simulink model "CH_humanoid_walker_rl"  (R2021a)
settings: Solver=daessc  StartTime=0.0  StopTime=params.simulation.Tf  RelTol=1e-3  AbsTol=1e-3
model workspace (MATLAB code in the model file):
  | %% Humanoid Walker With Reinforcement Learning Intialization
  | % Copyright 2019 The MathWorks, Inc.
  | 
  | %% Joint rotation limits
  | %These limits are similar to human joint rotation limits.
  | 
  | % Legs joints
  | params.jointLimits.hipFrontalUpperLimit  =  30;  % (Deg)
  | params.jointLimits.hipFrontalLowerLimit  = -90;  % (Deg)
  | params.jointLimits.kneeUpperLimit        =  90;  % (Deg)
  | params.jointLimits.kneeLowerLimit        =  5;   % (Deg)
  | params.jointLimits.ankleUpperLimit       =  20;  % (Deg)
  | params.jointLimits.ankleLowerLimit       = -20;  % (Deg)
  | % Arm joints
  | params.jointLimits.shoulderFrontalUpperLimit        =  110; % (Deg)
  | params.jointLimits.shoulderFrontalLowerLimit        = -30;  % (Deg)
  | params.jointLimits.shoulderSagittalUpperLimit       =  90;  % (Deg)
  | params.jointLimits.shoulderSagittalLowerLimit       = -30;  % (Deg)
  | params.jointLimits.elbowLowerLimit                  = 5;    % (Deg)
  | params.jointLimits.elbowUpperLimit                  = 130;  % (Deg)
  | params.jointLimits.wristLowerLimit                  = -90;  % (Deg)
  | params.jointLimits.wristUpperLimit                  = 70;   % (Deg)
  | 
  | %% Motor Parameters: Left
  | % Current motor: https://uk.rs-online.com/web/p/dc-motors/7736804
  | %Stall Torque
  | params.motor.StallTorque.LeftHip                        = 100; % (Nm)
  | params.motor.StallTorque.LeftKnee                       = 100; % (Nm)
  | params.motor.StallTorque.LeftAnkle                      = 100; % (Nm)
  | 
  | params.motor.StallTorque.LeftShoulderFrontal            = 100; % (Nm)
  | params.motor.StallTorque.LeftShoulderSagital            = 100; % (Nm)
  | params.motor.StallTorque.LeftElbow                      = 100; % (Nm)
  | params.motor.StallTorque.LeftWrist                      = 100; % (Nm)
  | 
  | %Armature Inductance: UNKNOWN
  | params.motor.ArmatureInductance.LeftHip                 = 12e-6;
  | params.motor.ArmatureInductance.LeftKnee                = 12e-6;
  | params.motor.ArmatureInductance.LeftAnkle               = 12e-6;
  | 
  | params.motor.ArmatureInductance.LeftShoulderFrontal     = 12e-6;
  | params.motor.ArmatureInductance.LeftShoulderSagital     = 12e-6;
  | params.motor.ArmatureInductance.LeftElbow               = 12e-6;
  | params.motor.ArmatureInductance.LeftWrist               = 12e-6;
  | 
  | %No-Load Speed
  | params.motor.NoLoadSpeed.LeftHip                        = 22.5; % (RPM)
  | params.motor.NoLoadSpeed.LeftKnee                       = 22.5; % (RPM)
  | params.motor.NoLoadSpeed.LeftAnkle                      = 22.5; % (RPM)
  | 
  | params.motor.NoLoadSpeed.LeftShoulderFrontal            = 22.5; % (RPM)
  | params.motor.NoLoadSpeed.LeftShoulderSagital            = 22.5; % (RPM)
  | params.motor.NoLoadSpeed.LeftElbow                      = 22.5; % (RPM)
  | params.motor.NoLoadSpeed.LeftWrist                      = 22.5; % (RPM)
  | 
  | %Torque Constant
  | params.motor.RatedDCSupply.LeftHip                      = 12; % (V)
  | params.motor.RatedDCSupply.LeftKnee                     = 12; % (V)
  | params.motor.RatedDCSupply.LeftAnkle                    = 12; % (V)
  | 
  | params.motor.RatedDCSupply.LeftShoulderFrontal          = 12; % (V)
  | params.motor.RatedDCSupply.LeftShoulderSagital          = 12; % (V)
  | params.motor.RatedDCSupply.LeftElbow                    = 12; % (V)
  | params.motor.RatedDCSupply.LeftWrist                    = 12; % (V)
  | 
  | %% Motor Parameters: Right
  | %Stall Torque
  | params.motor.StallTorque.RightHip                        = 100; % (Nm)
  | params.motor.StallTorque.RightKnee                       = 100; % (Nm)
  | params.motor.StallTorque.RightAnkle                      = 100; % (Nm)
  | 
  | params.motor.StallTorque.RightShoulderFrontal            = 100; % (Nm)
  | params.motor.StallTorque.RightShoulderSagital            = 100; % (Nm)
  | params.motor.StallTorque.RightElbow                      = 100; % (Nm)
  | params.motor.StallTorque.RightWrist                      = 100; % (Nm)
  | 
  | %Armature Inductance
  | params.motor.ArmatureInductance.RightHip                 = 12e-6;
  | params.motor.ArmatureInductance.RightKnee                = 12e-6;
  | params.motor.ArmatureInductance.RightAnkle               = 12e-6;
  | 
  | params.motor.ArmatureInductance.RightShoulderFrontal     = 12e-6;
  | params.motor.ArmatureInductance.RightShoulderSagital     = 12e-6;
  | params.motor.ArmatureInductance.RightElbow               = 12e-6;
  | params.motor.ArmatureInductance.RightWrist               = 12e-6;
  | 
  | %No-Load Speed
  | params.motor.NoLoadSpeed.RightHip                        = 22.5; % (RPM)
  | params.motor.NoLoadSpeed.RightKnee                       = 22.5; % (RPM)
  | params.motor.NoLoadSpeed.RightAnkle                      = 22.5; % (RPM)
  | 
  | params.motor.NoLoadSpeed.RightShoulderFrontal            = 22.5; % (RPM)
  | params.motor.NoLoadSpeed.RightShoulderSagital            = 22.5; % (RPM)
  | params.motor.NoLoadSpeed.RightElbow                      = 22.5; % (RPM)
  | params.motor.NoLoadSpeed.RightWrist                      = 22.5; % (RPM)
  | 
  | %Torque Constant
  | params.motor.RatedDCSupply.RightHip                      = 12; % (V)
  | params.motor.RatedDCSupply.RightKnee                     = 12; % (V)
  | params.motor.RatedDCSupply.RightAnkle                    = 12; % (V)
  | 
  | params.motor.RatedDCSupply.RightShoulderFrontal          = 12; % (V)
  | params.motor.RatedDCSupply.RightShoulderSagital          = 12; % (V)
  | params.motor.RatedDCSupply.RightElbow                    = 12; % (V)
  | params.motor.RatedDCSupply.RightWrist                    = 12; % (V)
  | 
  | 
  | %% Material properties
  | 
  | params.materialProperties.lowerBodyDensity = 990;  % (kg/m^3)
  | params.materialProperties.upperBodyDensity = 1900; % (kg/m^3)
  | 
  | %% World damping
  | % We add damping to the vertical (z) and rotational (Rx, Ry, Rz) components
  | % of the bushing joint. This dissipates energy from the system and facilates
  | % quicker learning. Increasing this improves stability and learning, but is
  | % less realistic.
  | 
  | params.simulation.worldDamping = 6; % (Ns/m)
  | 
  | %% Simulation parameters
  | 
  | params.simulation.initialHeight=1.54; % (m) Intial height of robot
  | params.simulation.Ts = 0.025;         % (s) Control and sensing discretization time
  | params.simulation.Tf = 600;      % (s) Max simulation time
  | 
  | %% Spatial contact force block parameters.
  | % The value of these parameters affects simulation and learning speed.
  | % Higher damping generally improves learning but slows down simulation.
  | % High static and dynamic friction values tend to improve learning.
  | 
  | params.contact.stiffness        = 1e5;  % (N/m)
  | params.contact.damping          = 1e5;  % (Ns/m)
  | params.contact.transitionWidth  = 1e-3; % (m)
  | params.contact.staticFriction   = 1;    % ()
  | params.contact.dynamicFriction  = 0.9;  % ()
  | params.contact.criticalVelocity = 1e-3; % (m/s)
  | params.contact.contactRadius = 0.01;    % (m)
  | 
  | %% Controller parameters
  | 
  | params.controller.hipFrontalStiffness  = 80; % (N*m/rad)
  | params.controller.hipFrontalDamping    = 1;  % (N*m*s/rad)
  | params.controller.kneeStiffness        = 80; % (N*m*/rad)
  | params.controller.kneeDamping          = 1;  % (N*m*s/rad)
  | params.controller.ankleStiffness       = 80; % (N*m/rad)
  | params.controller.ankleDamping         = 1;  % (N*m*s/rad)
  | 
  | 
  | %% Stopping criteria
  | % Define the conditions under which the simulation is terminated early.
  | % One or more of three conditions need to be satisfied for termination.
  | % If the humanoid torso drops vertically, travels laterally or rotates in
  | % any axis more than a set of predefined values, or if the humanoid stops
  | % moving.
  | 
  | params.stoppingCriteria.heightChange     = 0.5; % (m)
  | params.stoppingCriteria.lateral          = 1000;   % (m)
  | params.stoppingCriteria.angle            = 60;  % (deg)
  | params.stoppingCriteria.timeoutTime      = 2;   % (s)
  | params.stoppingCriteria.timeoutDistance  = 1;   % (m)
  | 
  | %% Reward scaling parameters
  | 
  | params.reward.boxMoveRewardWeight   = 5;    % Object motion reward scale, w_1
  | params.reward.forwardRewardWeight   = 1;    % Forward velocity scale, w_2
  | params.reward.timestepRewardWeight  = -0.5;    % Not falling scale, w_3 - Penalise time taken, Strive to always move forward
  | params.reward.powerPenaltyWeight    = 5e-4; % Power scale, w_4
  | params.reward.verticalPenaltyWeight = 25;   % Vertical displacement scale, w_5
  | params.reward.lateralPenaltyWeight  = 2;  % Lateral displacement scale, w_6
  | 
  | %% Display parameters
  | 
  | params.display.tileColour    = [0.956, 0.941, 0.941];
  | params.display.floorColour   = [0.756, 0.741, 0.741];
  | params.display.tileThickness = 0.005;
  | params.display.planeWidth        = 100;   % (m)
  | params.display.planeLength       = 200;  % (m)
  | params.display.planeHeight       = 1;   % (m)
  | params.display.Gravity           = [0, 0, -9.80665];   % (m/s^2)
undefined symbols (not defined in the file or in its folder): Connection1, Connection2, Connection3, Connection4, Connection5, Connection6, Connection7, Connection8, rl, X, Y, Z
libraries: sm_lib x26, CH_Library x8, nesl_utility x4, rllib x1
settings Model: Creator=The MathWorks, Inc.  LastModifiedBy=coa19cdd
settings SolverCC: AlgebraicLoopSolver=TrustRegion
settings DebuggingCC: ParameterPrecisionLossMsg=none  ParameterTunabilityLossMsg=none  SFMachineParentedDataDiag=warning
settings ExplorerConfigSet: InternalSimMechanicsExplorerSettings="<ExplorerConfiguration><canonicalview>default</canonicalview><AnimationSetting><BasePlaybackSpeed>1.0</BasePlaybackSpeed><PlaybackSpeedFactor>1.0</PlaybackSpeedFactor></AnimationSetting><TilePanel><TileInfo><Tiles Columns=\"1\" Count=\"1\" Rows=\"1\"><Column Weight=\"1\"/><Row Weight=\"1\"/><Tile Height=\"1\" Width=\"1\" X=\"0\" Y=\"0\"/></Tiles></TileInfo><SceneInfo><SceneViewer><BGColor><R>0.800000011920928955</R><G>1</G><B>1</B></BGColor><Camera><DoPerspective>on</DoPerspective><Position><X>41.8085971876439402</X><Y>-114.741449940210288</Y><Z>43.3892163501630179</Z></Position><Center><X>-86.6397285289506698</X><Y>13.7068757763843223</Y><Z>-85.0591093664316418</Z></Center><Up><X>-0.408248290463863073</X><Y>0.408248290463863073</Y><Z>0.816496580927726145</Z></Up><ViewLimDist>1</ViewLimDist><YLim>0.466307658154998583</YLim><XLim>0.727439946721797792</XLim></Camera></SceneViewer></SceneInfo></TilePanel><MechEditorPanel><Cameras><Camera><Id>Camera1</Id><Value><Name>Camera1</Name><NativeCamera><PositionTrackingFeature>Humanoid_Walker.Humanoid_Robot_6_Joint.Camera_Frame.R</PositionTrackingFeature><CenterTrackingFeature>Humanoid_Walker.Humanoid_Robot_6_Joint.Aim_Frame.R</CenterTrackingFeature><UpVectorTrackingFeature>Humanoid_Walker.Humanoid_Robot_6_Joint.World.W</UpVectorTrackingFeature><CenterTrackingOrigin>on</CenterTrackingOrigin><UpVectorTrackingDirection>+Z</UpVectorTrackingDirection></NativeCamera></Value></Camera></Cameras><GfxPanelCameraMap><MapElement CameraMLId=\"Camera1\" GfxPanelIndex=\"0\"/></GfxPanelCameraMap><VideoCreator><PlaybackSpeedRatio>1.0</PlaybackSpeedRatio><FrameRate>30</FrameRate><VideoFormat>Motion JPEG AVI</VideoFormat><FrameSize>auto</FrameSize></VideoCreator></MechEditorPanel></ExplorerConfiguration>"

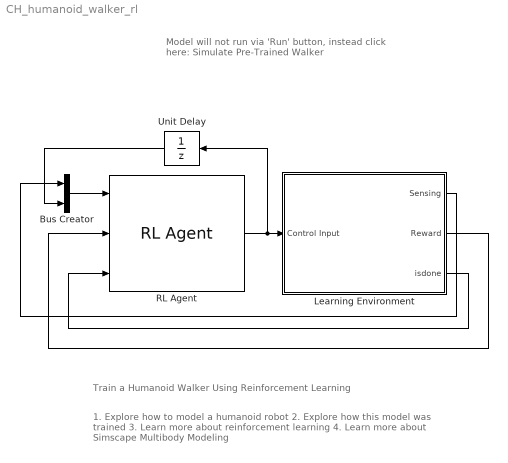
== system CH_humanoid_walker_rl ==
  note: Train a Humanoid Walker Using Reinforcement Learning
  note: Model will not run via 'Run' button, instead click here:
      | Simulate Pre-Trained Walker
  note: 1. Explore how to model a humanoid robot
      | 2. Explore how this model was trained
      | 3. Learn more about reinforcement learning
      | 4. Learn more about Simscape Multibody Modeling
  Bus Creator : BusCreator  Inputs=2
  Learning Environment : Subsystem
  RL Agent : rllib/RL Agent  Agent=rl.util.PolicyInstance.get()  ExternalActionAsInput=off  ProvideCumRwd=off  TreatAsDirectFeedthrough=on
  Unit Delay : UnitDelay  SampleTime=params.simulation.Ts  HasFrameUpgradeWarning=on
  wires:
  RL Agent/1 -> Unit Delay/1, Learning Environment/1(Control Input)
  Learning Environment/2("Reward ") -> RL Agent/2
  Learning Environment/3(isdone) -> RL Agent/3
  Bus Creator/1 -> RL Agent/1
  Unit Delay/1 -> Bus Creator/2
  Learning Environment/1(Sensing) -> Bus Creator/1

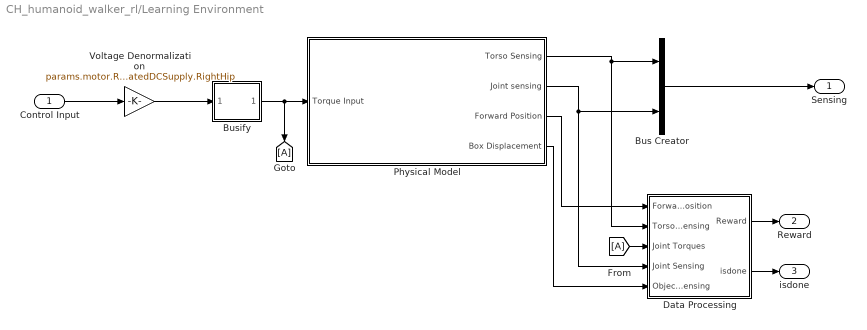
== system CH_humanoid_walker_rl/Learning Environment ==
  Control Input : Inport
  Bus Creator : BusCreator  Inputs=2
  Busify : Subsystem
  Data Processing : Subsystem
  Physical Model : Subsystem
  Voltage Denormalization : Gain  Gain=params.motor.RatedDCSupply.RightHip
  Sensing : Outport
  "Reward " : Outport  Port=2
  isdone : Outport  Port=3
  wires:
  Control Input/1 -> Voltage Denormalization/1
  Physical Model/1(Torso Sensing) -> Data Processing/2(Torso Sensing), Bus Creator/1
  Physical Model/2(Joint sensing) -> Data Processing/4(Joint Sensing), Bus Creator/2
  Busify/1(Out1) -> [A], Physical Model/1(Torque Input)
  [A] -> Data Processing/3(Joint Torques)
  Data Processing/1(Reward) -> "Reward "/1
  Data Processing/2(isdone) -> isdone/1
  Physical Model/3(Forward Position) -> Data Processing/1(Forward Position)
  Voltage Denormalization/1 -> Busify/1(Control Input)
  Bus Creator/1 -> Sensing/1
  Physical Model/4(Box Displacement) -> Data Processing/5(Object Sensing)

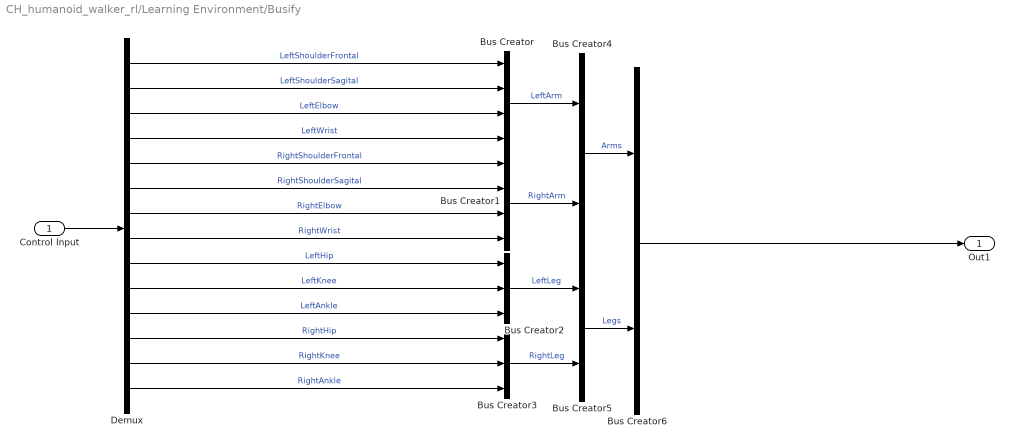
== system CH_humanoid_walker_rl/Learning Environment/Busify ==
  Control Input : Inport
  Bus Creator : BusCreator  Inputs=4
  Bus Creator1 : BusCreator  Inputs=4
  Bus Creator2 : BusCreator  Inputs=3
  Bus Creator3 : BusCreator  Inputs=3
  Bus Creator4 : BusCreator  Inputs=2
  Bus Creator5 : BusCreator  Inputs=2
  Bus Creator6 : BusCreator  Inputs=2
  Demux : Demux  Outputs=14
  Out1 : Outport
  wires:
  Control Input/1 -> Demux/1
  Demux/1 -> Bus Creator/1  "LeftShoulderFrontal"
  Demux/2 -> Bus Creator/2  "LeftShoulderSagital"
  Demux/3 -> Bus Creator/3  "LeftElbow"
  Demux/4 -> Bus Creator/4  "LeftWrist"
  Demux/5 -> Bus Creator1/1  "RightShoulderFrontal"
  Demux/6 -> Bus Creator1/2  "RightShoulderSagital"
  Demux/7 -> Bus Creator1/3  "RightElbow"
  Demux/8 -> Bus Creator1/4  "RightWrist"
  Demux/9 -> Bus Creator2/1  "LeftHip"
  Demux/10 -> Bus Creator2/2  "LeftKnee"
  Demux/11 -> Bus Creator2/3  "LeftAnkle"
  Demux/12 -> Bus Creator3/1  "RightHip"
  Demux/13 -> Bus Creator3/2  "RightKnee"
  Demux/14 -> Bus Creator3/3  "RightAnkle"
  Bus Creator/1 -> Bus Creator4/1  "LeftArm"
  Bus Creator1/1 -> Bus Creator4/2  "RightArm"
  Bus Creator2/1 -> Bus Creator5/1  "LeftLeg"
  Bus Creator3/1 -> Bus Creator5/2  "RightLeg"
  Bus Creator4/1 -> Bus Creator6/1  "Arms"
  Bus Creator5/1 -> Bus Creator6/2  "Legs"
  Bus Creator6/1 -> Out1/1

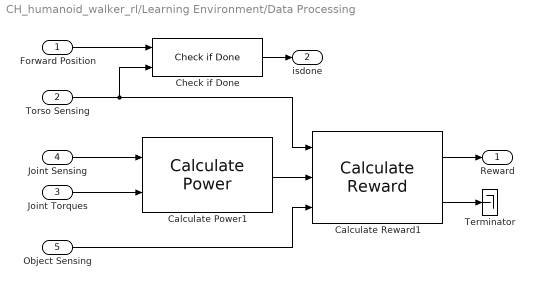
== system CH_humanoid_walker_rl/Learning Environment/Data Processing ==
  Forward Position : Inport
  Torso Sensing : Inport  Port=2
  Joint Torques : Inport  Port=3
  Joint Sensing : Inport  Port=4
  Object Sensing : Inport  Port=5
  Calculate Power1 : CH_Library/Calculate Power  SystemSampleTime=-1  VariantActivationTime=update diagram  Latency=0  AutoFrameSizeCalculation=off
  Calculate Reward1 : CH_Library/Calculate Reward  BoxReward=params.reward.boxMoveRewardWeight  forwardReward=params.reward.forwardRewardWeight  timestepReward=params.reward.timestepRewardWeight  powerPenalty=params.reward.powerPenaltyWeight  verticalPenalty=params.reward.verticalPenaltyWeight  lateralPenalty=params.reward.lateralPenaltyWeight
  Check if Done : CH_Library/Check if Done  verticalStop=params.stoppingCriteria.heightChange  lateralStop=params.stoppingCriteria.lateral  angularStop=params.stoppingCriteria.angle  timeoutTime=params.stoppingCriteria.timeoutTime  timeoutDistance=params.stoppingCriteria.timeoutDistance
  Terminator : Terminator
  Reward : Outport
  isdone : Outport  Port=2
  wires:
  Torso Sensing/1 -> Calculate Reward1/1, Check if Done/2
  Check if Done/1 -> isdone/1
  Calculate Power1/1 -> Calculate Reward1/2
  Joint Sensing/1 -> Calculate Power1/1
  Joint Torques/1 -> Calculate Power1/2
  Calculate Reward1/1 -> Reward/1
  Forward Position/1 -> Check if Done/1
  Calculate Reward1/2 -> Terminator/1
  Object Sensing/1 -> Calculate Reward1/3

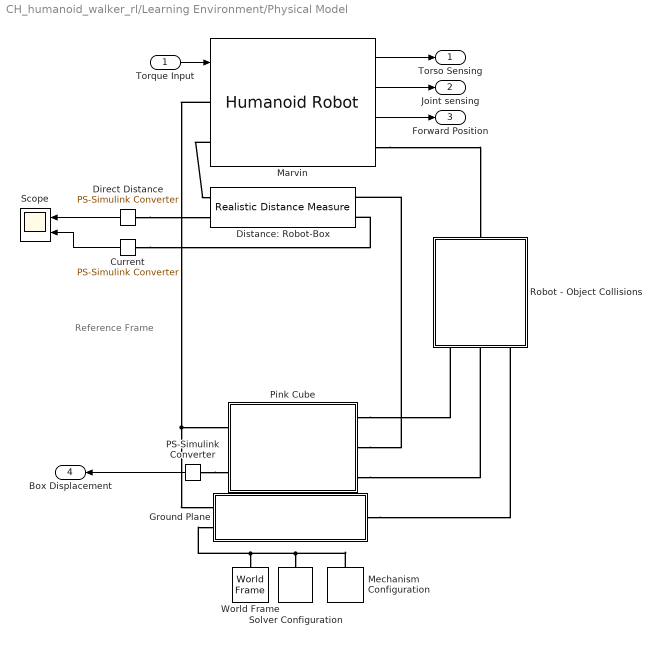
== system CH_humanoid_walker_rl/Learning Environment/Physical Model ==
  note: Reference Frame
  Torque Input : Inport
  Current : nesl_utility/PS-Simulink Converter  PhysicalDomain=network_engine_domain  SubClassName=ps_output  LeftPortType=input  RightPortType=output  PseudoPeriodic=off  Frequencies=[]  Unit=inherit  AffineConversion=off
      settings: SourceProductBaseCode=PW,SS
  Direct Distance : nesl_utility/PS-Simulink Converter  PhysicalDomain=network_engine_domain  SubClassName=ps_output  LeftPortType=input  RightPortType=output  PseudoPeriodic=off  Frequencies=[]  Unit=inherit  AffineConversion=off
      settings: SourceProductBaseCode=PW,SS
  Distance: Robot-Box : CH_Library/Realistic Distance Measure  LEDC=1.0
  Ground Plane : Subsystem
  Marvin : CH_Library/Humanoid Robot  contactRadius=params.contact.contactRadius  contactStiffness=params.contact.stiffness  contactDamping=params.contact.damping  contactTWidth=params.contact.transitionWidth  contactStaticFriction=params.contact.staticFriction  contactDynamicFriction=params.contact.dynamicFriction  contactCriticalVelocity=params.contact.criticalVelocity  footDensity=params.materialProperties.lowerBodyDensity  lowerLegDensity=params.materialProperties.lowerBodyDensity  upperLegDensity=params.materialProperties.lowerBodyDensity  hipDensity=params.materialProperties.lowerBodyDensity  trunkDensity=params.materialProperties.upperBodyDensity  shoulderDensity=params.materialProperties.upperBodyDensity  upperArmDensity=params.materialProperties.upperBodyDensity  lowerArmDensity=params.materialProperties.upperBodyDensity  handDensity=params.materialProperties.upperBodyDensity  headDensity=params.materialProperties.upperBodyDensity  hipUpperLimit=params.jointLimits.hipFrontalUpperLimit  hipLowerLimit=params.jointLimits.hipFrontalLowerLimit  kneeUpperLimit=params.jointLimits.kneeUpperLimit  kneeLowerLimit=params.jointLimits.kneeLowerLimit  ankleUpperLimit=params.jointLimits.ankleUpperLimit  ankleLowerLimit=params.jointLimits.ankleLowerLimit  shoulderFrontalUpperLimit=params.jointLimits.shoulderFrontalUpperLimit  shoulderFrontalLowerLimit=params.jointLimits.shoulderFrontalLowerLimit  shoulderSagittalUpperLimit=params.jointLimits.shoulderSagittalUpperLimit  shoulderSagittalLowerLimit=params.jointLimits.shoulderSagittalLowerLimit  elbowUpperLimit=params.jointLimits.ankleUpperLimit  elbowLowerLimit=params.jointLimits.shoulderSagittalLowerLimit  wristUpperLimit=params.jointLimits.ankleUpperLimit  wristLowerLimit=params.jointLimits.shoulderSagittalLowerLimit
      link override Torso and Head/Camera: Y_TF=5.0  X_ROT=10
  Mechanism Configuration : sm_lib/Utilities/Mechanism Configuration  UniformGravity=Constant  GravityVector=[0, 0, -9.80665]  GravityVectorUnits=m/s^2  GravityUnits=m/s^2  LinearizationDelta=0.001  JointModeTransitionNonlinearIterations=2
  PS-Simulink Converter : nesl_utility/PS-Simulink Converter  PhysicalDomain=network_engine_domain  SubClassName=ps_output  LeftPortType=input  RightPortType=output  PseudoPeriodic=off  Frequencies=[]  Unit=inherit  AffineConversion=off
      settings: SourceProductBaseCode=PW,SS
  Pink Cube : Subsystem  AncestorBlock=CH_Library/Brick Object Hybrid  mask{BW=1, BDep=1, BH=1, XDis=0, YDis=3, ZDis=0.6, XRot=0, YRot=0, ZRot=0, BDen=5, BlockRed=1.0, BlockGreen=0.680, BlockBlue=0.710, BlockOpac=1}
      mask prompts: BW "Width (X)"; BDep "Depth (Y)"; BH "Height (Z)"; XDis "X Displacement"; YDis "Y Displacement"; ZDis "Z Displacement"; XRot "Rotation about X"; YRot "Rotation about Y"; ZRot "Rotation about Z"; BDen "Density"; BlockRed "Red tint"; BlockGreen "Green tint"; BlockBlue "Blue tint"; BlockOpac "Opacity"
      mask DialogControl Container8 Prompt: Block Dimensions
      mask DialogControl Container11 Prompt: Block Placement
      mask DialogControl Container14 Prompt: Block Rotation
      mask DialogControl Control1 Prompt: Rotations completed in sequence: X,Y,Z
      mask DialogControl Container5 Prompt: Block Properties
  Robot - Object Collisions : Subsystem
      settings: PortSchema="{\"entries\":[{\"content\":{\"sides\":[{\"content\":{\"connectorIds\":[]},\"type\":\"ConnectorPlacement.EquallySpacedRectSide\",\"uuid\":\"b00614a5-f09e-422d-bac9-77beaa757f34\"},{\"content\":{\"connectorIds\":[],\"side\":\"RIGHT\"},\"type\":\"ConnectorPlacement.EquallySpacedRectSide\",\"uuid\":\"f8121b2f-8181-47c9-add5-f5a413d142f6\"},{\"content\":{\"connectorIds\":[\"LConn1\"],\"side\":\"TOP\"},\"type\":\"ConnectorPlacement.EquallySpacedRectSide\",\"uuid\":\"8b595efc-2aff-4bc7-847e-9a9432c1292e\"},{\"content\":{\"connectorIds\":[\"RConn1\",\"RConn2\",\"RConn3\"],\"side\":\"BOTTOM\"},\"type\":\"ConnectorPlacement.EquallySpacedRectSide\",\"uuid\":\"30d4c700-0653-4c9a-a829-31e4e720a8eb\"}]},\"type\":\"ConnectorPlacement.EquallySpacedConnector\",\"uuid\":\"6d11a0b2-f15b-484e-9b2d-8ecd8f664af7\"}],\"packageUris\":[\"http://schema.mathworks.com/mf0/Connector/R2020b\"],\"version\":\"1.0\"}"
  Scope : Scope  NumInputPorts=2
  Solver Configuration : nesl_utility/Solver Configuration  PhysicalDomain=network_engine_domain  SubClassName=solver  LeftPortType=input  RightPortType=generic  Tones=[]  Harmonics=[]  SimulateNoise=off  Profile=off  UseLocalSampling=off  EnableSwitchedLinearOptims=on  FrequencyDomain=off  UseCCode=off  RelTol=0.001  AbsTol=1e-06  MinStep=1e-09  ToWorkspace=off  RevertToSquareIcSolve=off  NumHomotopyIterations=100  PhasorMode=off  PhasorModeNumHarmonics=1  DoDC=off  ResidualTolerance=1e-09  UseLocalSolver=off  LocalSolverChoice=NE_BACKWARD_EULER_ADVANCER  LocalSolverSampleTime=0.001  DoFixedCost=off  MaxNonlinIter=3  MaxModeIter=2  ComputeImpulses=off  ImpulseIterations=2  LinearAlgebra=auto  EquationFormulation=NE_TIME_EF  DelaysMemoryBudget=1024  AutomaticFiltering=on  FilteringTimeConstant=0.001  PartitionStorageMethod=AS_NEEDED  PartitionMemoryBudget=1024  PartitionMethod=ROBUST
      settings: SourceProductBaseCode=PW,SS
  World Frame : sm_lib/Frames and Transforms/World Frame
  Torso Sensing : Outport
  Joint sensing : Outport  Port=2
  Forward Position : Outport  Port=3
  Box Displacement : Outport  Port=4
  wires:
  Torque Input/1 -> Marvin/1
  Marvin/3 -> Forward Position/1
  Marvin/2 -> Joint sensing/1
  Marvin/1 -> Torso Sensing/1
  Current/1 -> Scope/2
  Direct Distance/1 -> Scope/1
  PS-Simulink Converter/1 -> Box Displacement/1
  connections:
  Mechanism Configuration/RConn1 -- World Frame/RConn1 -- Ground Plane/LConn2 -- Solver Configuration/RConn1
  Marvin/LConn1 -- Pink Cube/LConn1 -- Ground Plane/LConn1
  Marvin/LConn2 -- Distance: Robot-Box/LConn1
  Pink Cube/RConn2 -- Distance: Robot-Box/RConn1
  Current/LConn1 -- Distance: Robot-Box/RConn2
  Direct Distance/LConn1 -- Distance: Robot-Box/LConn2
  Marvin/RConn1 -- Robot - Object Collisions/LConn1
  Ground Plane/RConn1 -- Robot - Object Collisions/RConn3
  Pink Cube/RConn1 -- Robot - Object Collisions/RConn1
  PS-Simulink Converter/LConn1 -- Pink Cube/LConn2
  Pink Cube/RConn3 -- Robot - Object Collisions/RConn2

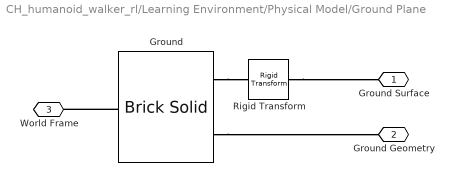
== system CH_humanoid_walker_rl/Learning Environment/Physical Model/Ground Plane ==
  Ground : sm_lib/Body Elements/Brick Solid  GraphicAmbientColor=[0.15 0.15 0.15 1.0]  BasedOnType=Density  BrickDimensions=[params.display.planeWidth params.display.planeLength params.display.planeHeight]  BrickDimensionUnits=m  CenterOfMass=[0 0 0]  CenterOfMassUnits=m  GraphicDiffuseColor=params.display.floorColour  Density=1000  DensityUnits=kg/m^3  DoExposeReferenceFrame=on  GraphicEmissiveColor=[0.0 0.0 0.0 1.0]  ExportEntireGeometry=on  SerializedFrames=<Frames><Frame><Id>Frame1</Id><Value><Name>GS</Name><Origin><Source>GeometricFeature</Source><FeatureName>+z surface</FeatureName></Origin><PrimaryAxis><DefinedDirection>+Z</DefinedDirection><Source>ReferenceFrame</Source><SourceDirection>+Z</SourceDirection><FeatureName></FeatureName></PrimaryAxis><SecondaryAxis><DefinedDirection>+X</DefinedDirection><Source>ReferenceFrame</Source><SourceDirection>+X</SourceDirection><FeatureName></FeatureName></SecondaryAxis></Value></Frame></Frames>  MarkerShape=Sphere  MarkerSize=10  GraphicType=FromGeometry  InertiaType=CalculateFromGeometry  Mass=1  MassUnits=kg  MomentsOfInertia=[1 1 1]  MomentsOfInertiaUnits=kg*m^2  GraphicOpacity=0.3  ProductsOfInertia=[0 0 0]  ProductsOfInertiaUnits=kg*m^2  GraphicShininess=75  GraphicSpecularColor=[0.5 0.5 0.5 1.0]  GraphicVisPropType=SimpleVisualProperties
  Rigid Transform : sm_lib/Frames and Transforms/Rigid Transform  TranslationMethod=StandardAxis  TranslationStandardOffset=0.5-(params.display.planeLength/2)  TranslationLengthUnit=m  TranslationStandardAxis=+Y  TranslationCartesianOffset=[0 0 0]  TranslationROffset=0  TranslationROffsetUnits=m  TranslationZOffset=0  TranslationZOffsetUnits=m  TranslationThetaOffset=0  TranslationThetaOffsetUnits=deg  RotationMethod=None  RotationAngleUnits=deg  RotationStandardAxis=+Z  RotationAngle=0.0  RotationArbitraryAxis=[0 0 1]  FollAlignAxisA=+X  BaseAlignAxisA=+Y  FollAlignAxisB=+Y  BaseAlignAxisB=+Z  RotationSequenceAxes=FollowerAxes  RotationSequence=XYX  RotationSequenceAngles=[0 0 0]  RotationSequenceAnglesUnits=deg  RotationMatrix=[1 0 0; 0 1 0; 0 0 1]
  Ground Surface : PMIOPort  Side=Left
  Ground Geometry : PMIOPort  Port=2  Side=Right
  World Frame : PMIOPort  Port=3  Side=Left
  connections:
  Ground/LConn1 -- Rigid Transform/LConn1
  Ground/LConn2 -- Ground Geometry/RConn1
  Ground/RConn1 -- World Frame/RConn1
  Rigid Transform/RConn1 -- Ground Surface/RConn1

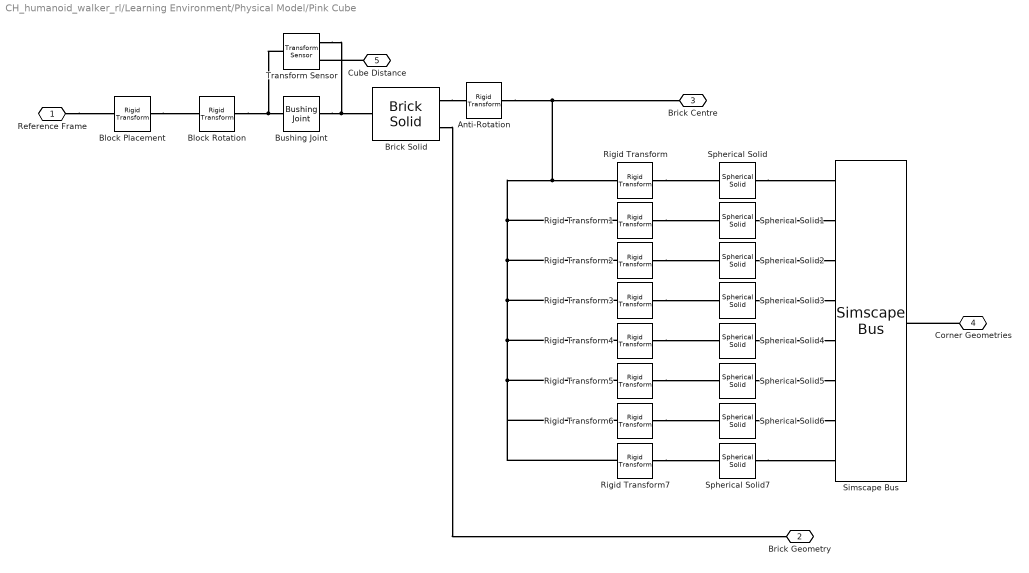
== system CH_humanoid_walker_rl/Learning Environment/Physical Model/Pink Cube ==
  Anti-Rotation : sm_lib/Frames and Transforms/Rigid Transform  TranslationMethod=None  TranslationStandardOffset=0  TranslationLengthUnit=m  TranslationStandardAxis=+Z  TranslationCartesianOffset=[0 0 0]  TranslationROffset=0  TranslationROffsetUnits=m  TranslationZOffset=0  TranslationZOffsetUnits=m  TranslationThetaOffset=0  TranslationThetaOffsetUnits=deg  RotationMethod=RotationSequence  RotationAngleUnits=deg  RotationStandardAxis=+Z  RotationAngle=0.0  RotationArbitraryAxis=[0 0 1]  FollAlignAxisA=+X  BaseAlignAxisA=+Y  FollAlignAxisB=+Y  BaseAlignAxisB=+Z  RotationSequenceAxes=BaseAxes  RotationSequence=XYZ  RotationSequenceAngles=[-XRot -YRot -ZRot]  RotationSequenceAnglesUnits=deg  RotationMatrix=[1 0 0; 0 1 0; 0 0 1]
  Block Placement : sm_lib/Frames and Transforms/Rigid Transform  TranslationMethod=Cartesian  TranslationStandardOffset=0  TranslationLengthUnit=m  TranslationStandardAxis=+Z  TranslationCartesianOffset=[XDis YDis ZDis]  TranslationROffset=0  TranslationROffsetUnits=m  TranslationZOffset=0  TranslationZOffsetUnits=m  TranslationThetaOffset=0  TranslationThetaOffsetUnits=deg  RotationMethod=None  RotationAngleUnits=deg  RotationStandardAxis=+Z  RotationAngle=0.0  RotationArbitraryAxis=[0 0 1]  FollAlignAxisA=+X  BaseAlignAxisA=+Y  FollAlignAxisB=+Y  BaseAlignAxisB=+Z  RotationSequenceAxes=FollowerAxes  RotationSequence=XYX  RotationSequenceAngles=[0 0 0]  RotationSequenceAnglesUnits=deg  RotationMatrix=[1 0 0; 0 1 0; 0 0 1]
  Block Rotation : sm_lib/Frames and Transforms/Rigid Transform  TranslationMethod=None  TranslationStandardOffset=0  TranslationLengthUnit=m  TranslationStandardAxis=+Z  TranslationCartesianOffset=[0 0 0]  TranslationROffset=0  TranslationROffsetUnits=m  TranslationZOffset=0  TranslationZOffsetUnits=m  TranslationThetaOffset=0  TranslationThetaOffsetUnits=deg  RotationMethod=RotationSequence  RotationAngleUnits=deg  RotationStandardAxis=+Z  RotationAngle=0.0  RotationArbitraryAxis=[0 0 1]  FollAlignAxisA=+X  BaseAlignAxisA=+Y  FollAlignAxisB=+Y  BaseAlignAxisB=+Z  RotationSequenceAxes=BaseAxes  RotationSequence=XYZ  RotationSequenceAngles=[XRot YRot ZRot]  RotationSequenceAnglesUnits=deg  RotationMatrix=[1 0 0; 0 1 0; 0 0 1]
  Brick Solid : sm_lib/Body Elements/Brick Solid  GraphicAmbientColor=[0.15 0.15 0.15 1.0]  BasedOnType=Density  BrickDimensions=[BW BDep BH]  BrickDimensionUnits=m  CenterOfMass=[0 0 0]  CenterOfMassUnits=m  GraphicDiffuseColor=[BlockRed BlockGreen BlockBlue]  Density=BDen  DensityUnits=kg/m^3  DoExposeReferenceFrame=on  GraphicEmissiveColor=[0.0 0.0 0.0 1.0]  ExportEntireGeometry=on  SerializedFrames=<Frames><Frame><Id>Frame1</Id><Value><Name>Block Centre</Name><Origin><Source>ReferenceFrame</Source><FeatureName></FeatureName></Origin><PrimaryAxis><DefinedDirection>+Z</DefinedDirection><Source>ReferenceFrame</Source><SourceDirection>+Z</SourceDirection><FeatureName></FeatureName></PrimaryAxis><SecondaryAxis><DefinedDirection>+X</DefinedDirection><Source>ReferenceFrame</Source><SourceDirection>+X</SourceDirection><FeatureName></FeatureName></SecondaryAxis></Value></Frame></Frames>  MarkerShape=Sphere  MarkerSize=10  GraphicType=FromGeometry  InertiaType=CalculateFromGeometry  Mass=1  MassUnits=kg  MomentsOfInertia=[1 1 1]  MomentsOfInertiaUnits=kg*m^2  GraphicOpacity=BlockOpac  ProductsOfInertia=[0 0 0]  ProductsOfInertiaUnits=kg*m^2  GraphicShininess=75  GraphicSpecularColor=[0.5 0.5 0.5 1.0]  GraphicVisPropType=SimpleVisualProperties
  Bushing Joint : sm_lib/Joints/Bushing Joint  JointMode=Normal  SenseConstraintForce=off  SenseConstraintForceX=off  SenseConstraintForceY=off  SenseConstraintForceZ=off  SenseConstraintTorque=off  SenseConstraintTorqueX=off  SenseConstraintTorqueY=off  SenseConstraintTorqueZ=off  SenseTotalForce=off  SenseTotalForceX=off  SenseTotalForceY=off  SenseTotalForceZ=off  SenseTotalTorque=off  SenseTotalTorqueX=off  SenseTotalTorqueY=off  SenseTotalTorqueZ=off  CompositeWrenchDir=FollowerOnBase  CompositeWrenchFrame=BaseFrame  PxEquilibriumPosition=0  PxEquilibriumPositionUnits=m  PxSpringStiffness=0  PxSpringStiffnessUnits=N/m  PxDampingCoefficient=0  PxDampingCoefficientUnits=N/(m/s)  PxTorqueActuationMode=NoTorque  PxMotionActuationMode=ComputedMotion  PxSensePosition=off  PxSenseVelocity=off  PxSenseAcceleration=off  PxSenseTorqueForce=off  PxSenseLowerLimitTorqueForce=off  PxSenseUpperLimitTorqueForce=off  PxLowerLimitSpecify=off  PxLowerLimitBound=-1  PxLowerLimitBoundUnits=m  PxLowerLimitStiffness=1e6  PxLowerLimitStiffnessUnits=N/m  PxLowerLimitDamping=1e3  PxLowerLimitDampingUnits=N/(m/s)  PxLowerLimitTransitionRegionWidth=1e-4  PxLowerLimitTransitionRegionWidthUnits=m  PxUpperLimitSpecify=off  PxUpperLimitBound=1  PxUpperLimitBoundUnits=m  PxUpperLimitStiffness=1e6  PxUpperLimitStiffnessUnits=N/m  PxUpperLimitDamping=1e3  PxUpperLimitDampingUnits=N/(m/s)  PxUpperLimitTransitionRegionWidth=1e-4  PxUpperLimitTransitionRegionWidthUnits=m  PxPositionTargetSpecify=off  PxPositionTargetPriority=High  PxPositionTargetValue=0  PxPositionTargetValueUnits=m  PxVelocityTargetSpecify=off  PxVelocityTargetPriority=High  PxVelocityTargetValue=0  PxVelocityTargetValueUnits=m/s  PyEquilibriumPosition=0  PyEquilibriumPositionUnits=m  PySpringStiffness=0  PySpringStiffnessUnits=N/m  PyDampingCoefficient=0  PyDampingCoefficientUnits=N/(m/s)  PyTorqueActuationMode=NoTorque  PyMotionActuationMode=ComputedMotion  PySensePosition=off  PySenseVelocity=off  PySenseAcceleration=off  PySenseTorqueForce=off  PySenseLowerLimitTorqueForce=off  PySenseUpperLimitTorqueForce=off  PyLowerLimitSpecify=off  PyLowerLimitBound=-1  PyLowerLimitBoundUnits=m  PyLowerLimitStiffness=1e6  PyLowerLimitStiffnessUnits=N/m  PyLowerLimitDamping=1e3  PyLowerLimitDampingUnits=N/(m/s)  PyLowerLimitTransitionRegionWidth=1e-4  PyLowerLimitTransitionRegionWidthUnits=m  PyUpperLimitSpecify=off  PyUpperLimitBound=1  PyUpperLimitBoundUnits=m  PyUpperLimitStiffness=1e6  PyUpperLimitStiffnessUnits=N/m  PyUpperLimitDamping=1e3  PyUpperLimitDampingUnits=N/(m/s)  PyUpperLimitTransitionRegionWidth=1e-4  PyUpperLimitTransitionRegionWidthUnits=m  PyPositionTargetSpecify=off  PyPositionTargetPriority=High  PyPositionTargetValue=0  PyPositionTargetValueUnits=m  PyVelocityTargetSpecify=off  PyVelocityTargetPriority=High  PyVelocityTargetValue=0  PyVelocityTargetValueUnits=m/s  PzEquilibriumPosition=0  PzEquilibriumPositionUnits=m  PzSpringStiffness=0  PzSpringStiffnessUnits=N/m  PzDampingCoefficient=0  PzDampingCoefficientUnits=N/(m/s)  PzTorqueActuationMode=NoTorque  PzMotionActuationMode=ComputedMotion  PzSensePosition=off  PzSenseVelocity=off  PzSenseAcceleration=off  PzSenseTorqueForce=off  PzSenseLowerLimitTorqueForce=off  PzSenseUpperLimitTorqueForce=off  PzLowerLimitSpecify=off  PzLowerLimitBound=-1  PzLowerLimitBoundUnits=m  PzLowerLimitStiffness=1e6  PzLowerLimitStiffnessUnits=N/m  PzLowerLimitDamping=1e3  PzLowerLimitDampingUnits=N/(m/s)  PzLowerLimitTransitionRegionWidth=1e-4  PzLowerLimitTransitionRegionWidthUnits=m  PzUpperLimitSpecify=off  PzUpperLimitBound=1  PzUpperLimitBoundUnits=m  PzUpperLimitStiffness=1e6  PzUpperLimitStiffnessUnits=N/m  PzUpperLimitDamping=1e3  PzUpperLimitDampingUnits=N/(m/s)  PzUpperLimitTransitionRegionWidth=1e-4  PzUpperLimitTransitionRegionWidthUnits=m  PzPositionTargetSpecify=off  PzPositionTargetPriority=High  PzPositionTargetValue=0  PzPositionTargetValueUnits=m  PzVelocityTargetSpecify=off  PzVelocityTargetPriority=High  PzVelocityTargetValue=0  PzVelocityTargetValueUnits=m/s  RxEquilibriumPosition=0  RxEquilibriumPositionUnits=deg  RxSpringStiffness=0  RxSpringStiffnessUnits=N*m/deg  RxDampingCoefficient=0  RxDampingCoefficientUnits=N*m/(deg/s)  RxTorqueActuationMode=NoTorque  RxMotionActuationMode=ComputedMotion  RxSensePosition=off  RxSenseVelocity=off  RxSenseAcceleration=off  RxSenseTorqueForce=off  RxSenseLowerLimitTorqueForce=off  RxSenseUpperLimitTorqueForce=off  RxLowerLimitSpecify=off  RxLowerLimitBound=-90  RxLowerLimitBoundUnits=deg  RxLowerLimitStiffness=1e4  RxLowerLimitStiffnessUnits=N*m/deg  RxLowerLimitDamping=10  RxLowerLimitDampingUnits=N*m/(deg/s)  RxLowerLimitTransitionRegionWidth=0.1  RxLowerLimitTransitionRegionWidthUnits=deg  RxUpperLimitSpecify=off  RxUpperLimitBound=90  RxUpperLimitBoundUnits=deg  RxUpperLimitStiffness=1e4  RxUpperLimitStiffnessUnits=N*m/deg  RxUpperLimitDamping=10  RxUpperLimitDampingUnits=N*m/(deg/s)  RxUpperLimitTransitionRegionWidth=0.1  RxUpperLimitTransitionRegionWidthUnits=deg  RxPositionTargetSpecify=off  RxPositionTargetPriority=High  RxPositionTargetValue=0  RxPositionTargetValueUnits=deg  RxVelocityTargetSpecify=off  RxVelocityTargetPriority=High  RxVelocityTargetValue=0  RxVelocityTargetValueUnits=deg/s  RyEquilibriumPosition=0  RyEquilibriumPositionUnits=deg  RySpringStiffness=0  RySpringStiffnessUnits=N*m/deg  RyDampingCoefficient=0  RyDampingCoefficientUnits=N*m/(deg/s)  RyTorqueActuationMode=NoTorque  RyMotionActuationMode=ComputedMotion  RySensePosition=off  RySenseVelocity=off  RySenseAcceleration=off  RySenseTorqueForce=off  RySenseLowerLimitTorqueForce=off  RySenseUpperLimitTorqueForce=off  RyLowerLimitSpecify=off  RyLowerLimitBound=-90  RyLowerLimitBoundUnits=deg  RyLowerLimitStiffness=1e4  RyLowerLimitStiffnessUnits=N*m/deg  RyLowerLimitDamping=10  RyLowerLimitDampingUnits=N*m/(deg/s)  RyLowerLimitTransitionRegionWidth=0.1  RyLowerLimitTransitionRegionWidthUnits=deg  RyUpperLimitSpecify=off  RyUpperLimitBound=90  RyUpperLimitBoundUnits=deg  RyUpperLimitStiffness=1e4  RyUpperLimitStiffnessUnits=N*m/deg  RyUpperLimitDamping=10  RyUpperLimitDampingUnits=N*m/(deg/s)  RyUpperLimitTransitionRegionWidth=0.1  RyUpperLimitTransitionRegionWidthUnits=deg  RyPositionTargetSpecify=off  RyPositionTargetPriority=High  RyPositionTargetValue=0  RyPositionTargetValueUnits=deg  RyVelocityTargetSpecify=off  RyVelocityTargetPriority=High  RyVelocityTargetValue=0  RyVelocityTargetValueUnits=deg/s  RzEquilibriumPosition=0  RzEquilibriumPositionUnits=deg  RzSpringStiffness=0  RzSpringStiffnessUnits=N*m/deg  RzDampingCoefficient=0  RzDampingCoefficientUnits=N*m/(deg/s)  RzTorqueActuationMode=NoTorque  RzMotionActuationMode=ComputedMotion  RzSensePosition=off  RzSenseVelocity=off  RzSenseAcceleration=off  RzSenseTorqueForce=off  RzSenseLowerLimitTorqueForce=off  RzSenseUpperLimitTorqueForce=off  RzLowerLimitSpecify=off  RzLowerLimitBound=-90  RzLowerLimitBoundUnits=deg  RzLowerLimitStiffness=1e4  RzLowerLimitStiffnessUnits=N*m/deg  RzLowerLimitDamping=10  RzLowerLimitDampingUnits=N*m/(deg/s)  RzLowerLimitTransitionRegionWidth=0.1  RzLowerLimitTransitionRegionWidthUnits=deg  RzUpperLimitSpecify=off  RzUpperLimitBound=90  RzUpperLimitBoundUnits=deg  RzUpperLimitStiffness=1e4  RzUpperLimitStiffnessUnits=N*m/deg  RzUpperLimitDamping=10  RzUpperLimitDampingUnits=N*m/(deg/s)  RzUpperLimitTransitionRegionWidth=0.1  RzUpperLimitTransitionRegionWidthUnits=deg  RzPositionTargetSpecify=off  RzPositionTargetPriority=High  RzPositionTargetValue=0  RzPositionTargetValueUnits=deg  RzVelocityTargetSpecify=off  RzVelocityTargetPriority=High  RzVelocityTargetValue=0  RzVelocityTargetValueUnits=deg/s
  Rigid Transform : sm_lib/Frames and Transforms/Rigid Transform  TranslationMethod=Cartesian  TranslationStandardOffset=0  TranslationLengthUnit=m  TranslationStandardAxis=+Z  TranslationCartesianOffset=[BW BH BDep]/2  TranslationROffset=0  TranslationROffsetUnits=m  TranslationZOffset=0  TranslationZOffsetUnits=m  TranslationThetaOffset=0  TranslationThetaOffsetUnits=deg  RotationMethod=None  RotationAngleUnits=deg  RotationStandardAxis=+Z  RotationAngle=0.0  RotationArbitraryAxis=[0 0 1]  FollAlignAxisA=+X  BaseAlignAxisA=+Y  FollAlignAxisB=+Y  BaseAlignAxisB=+Z  RotationSequenceAxes=FollowerAxes  RotationSequence=XYX  RotationSequenceAngles=[0 0 0]  RotationSequenceAnglesUnits=deg  RotationMatrix=[1 0 0; 0 1 0; 0 0 1]
  Rigid Transform1 : sm_lib/Frames and Transforms/Rigid Transform  TranslationMethod=Cartesian  TranslationStandardOffset=0  TranslationLengthUnit=m  TranslationStandardAxis=+Z  TranslationCartesianOffset=[BW BH -BDep]/2  TranslationROffset=0  TranslationROffsetUnits=m  TranslationZOffset=0  TranslationZOffsetUnits=m  TranslationThetaOffset=0  TranslationThetaOffsetUnits=deg  RotationMethod=None  RotationAngleUnits=deg  RotationStandardAxis=+Z  RotationAngle=0.0  RotationArbitraryAxis=[0 0 1]  FollAlignAxisA=+X  BaseAlignAxisA=+Y  FollAlignAxisB=+Y  BaseAlignAxisB=+Z  RotationSequenceAxes=FollowerAxes  RotationSequence=XYX  RotationSequenceAngles=[0 0 0]  RotationSequenceAnglesUnits=deg  RotationMatrix=[1 0 0; 0 1 0; 0 0 1]
  Rigid Transform2 : sm_lib/Frames and Transforms/Rigid Transform  TranslationMethod=Cartesian  TranslationStandardOffset=0  TranslationLengthUnit=m  TranslationStandardAxis=+Z  TranslationCartesianOffset=[BW -BH BDep]/2  TranslationROffset=0  TranslationROffsetUnits=m  TranslationZOffset=0  TranslationZOffsetUnits=m  TranslationThetaOffset=0  TranslationThetaOffsetUnits=deg  RotationMethod=None  RotationAngleUnits=deg  RotationStandardAxis=+Z  RotationAngle=0.0  RotationArbitraryAxis=[0 0 1]  FollAlignAxisA=+X  BaseAlignAxisA=+Y  FollAlignAxisB=+Y  BaseAlignAxisB=+Z  RotationSequenceAxes=FollowerAxes  RotationSequence=XYX  RotationSequenceAngles=[0 0 0]  RotationSequenceAnglesUnits=deg  RotationMatrix=[1 0 0; 0 1 0; 0 0 1]
  Rigid Transform3 : sm_lib/Frames and Transforms/Rigid Transform  TranslationMethod=Cartesian  TranslationStandardOffset=0  TranslationLengthUnit=m  TranslationStandardAxis=+Z  TranslationCartesianOffset=[BW -BH -BDep]/2  TranslationROffset=0  TranslationROffsetUnits=m  TranslationZOffset=0  TranslationZOffsetUnits=m  TranslationThetaOffset=0  TranslationThetaOffsetUnits=deg  RotationMethod=None  RotationAngleUnits=deg  RotationStandardAxis=+Z  RotationAngle=0.0  RotationArbitraryAxis=[0 0 1]  FollAlignAxisA=+X  BaseAlignAxisA=+Y  FollAlignAxisB=+Y  BaseAlignAxisB=+Z  RotationSequenceAxes=FollowerAxes  RotationSequence=XYX  RotationSequenceAngles=[0 0 0]  RotationSequenceAnglesUnits=deg  RotationMatrix=[1 0 0; 0 1 0; 0 0 1]
  Rigid Transform4 : sm_lib/Frames and Transforms/Rigid Transform  TranslationMethod=Cartesian  TranslationStandardOffset=0  TranslationLengthUnit=m  TranslationStandardAxis=+Z  TranslationCartesianOffset=[-BW BH BDep]/2  TranslationROffset=0  TranslationROffsetUnits=m  TranslationZOffset=0  TranslationZOffsetUnits=m  TranslationThetaOffset=0  TranslationThetaOffsetUnits=deg  RotationMethod=None  RotationAngleUnits=deg  RotationStandardAxis=+Z  RotationAngle=0.0  RotationArbitraryAxis=[0 0 1]  FollAlignAxisA=+X  BaseAlignAxisA=+Y  FollAlignAxisB=+Y  BaseAlignAxisB=+Z  RotationSequenceAxes=FollowerAxes  RotationSequence=XYX  RotationSequenceAngles=[0 0 0]  RotationSequenceAnglesUnits=deg  RotationMatrix=[1 0 0; 0 1 0; 0 0 1]
  Rigid Transform5 : sm_lib/Frames and Transforms/Rigid Transform  TranslationMethod=Cartesian  TranslationStandardOffset=0  TranslationLengthUnit=m  TranslationStandardAxis=+Z  TranslationCartesianOffset=[-BW BH -BDep]/2  TranslationROffset=0  TranslationROffsetUnits=m  TranslationZOffset=0  TranslationZOffsetUnits=m  TranslationThetaOffset=0  TranslationThetaOffsetUnits=deg  RotationMethod=None  RotationAngleUnits=deg  RotationStandardAxis=+Z  RotationAngle=0.0  RotationArbitraryAxis=[0 0 1]  FollAlignAxisA=+X  BaseAlignAxisA=+Y  FollAlignAxisB=+Y  BaseAlignAxisB=+Z  RotationSequenceAxes=FollowerAxes  RotationSequence=XYX  RotationSequenceAngles=[0 0 0]  RotationSequenceAnglesUnits=deg  RotationMatrix=[1 0 0; 0 1 0; 0 0 1]
  Rigid Transform6 : sm_lib/Frames and Transforms/Rigid Transform  TranslationMethod=Cartesian  TranslationStandardOffset=0  TranslationLengthUnit=m  TranslationStandardAxis=+Z  TranslationCartesianOffset=[-BW -BH BDep]/2  TranslationROffset=0  TranslationROffsetUnits=m  TranslationZOffset=0  TranslationZOffsetUnits=m  TranslationThetaOffset=0  TranslationThetaOffsetUnits=deg  RotationMethod=None  RotationAngleUnits=deg  RotationStandardAxis=+Z  RotationAngle=0.0  RotationArbitraryAxis=[0 0 1]  FollAlignAxisA=+X  BaseAlignAxisA=+Y  FollAlignAxisB=+Y  BaseAlignAxisB=+Z  RotationSequenceAxes=FollowerAxes  RotationSequence=XYX  RotationSequenceAngles=[0 0 0]  RotationSequenceAnglesUnits=deg  RotationMatrix=[1 0 0; 0 1 0; 0 0 1]
  Rigid Transform7 : sm_lib/Frames and Transforms/Rigid Transform  TranslationMethod=Cartesian  TranslationStandardOffset=0  TranslationLengthUnit=m  TranslationStandardAxis=+Z  TranslationCartesianOffset=[-BW -BH -BDep]/2  TranslationROffset=0  TranslationROffsetUnits=m  TranslationZOffset=0  TranslationZOffsetUnits=m  TranslationThetaOffset=0  TranslationThetaOffsetUnits=deg  RotationMethod=None  RotationAngleUnits=deg  RotationStandardAxis=+Z  RotationAngle=0.0  RotationArbitraryAxis=[0 0 1]  FollAlignAxisA=+X  BaseAlignAxisA=+Y  FollAlignAxisB=+Y  BaseAlignAxisB=+Z  RotationSequenceAxes=FollowerAxes  RotationSequence=XYX  RotationSequenceAngles=[0 0 0]  RotationSequenceAnglesUnits=deg  RotationMatrix=[1 0 0; 0 1 0; 0 0 1]
  Simscape Bus : SimscapeBus  HierarchyStrings=Connection1;Connection2;Connection3;Connection4;Connection5;Connection6;Connection7;Connection8
  Spherical Solid{,1..7} (8 alike) : sm_lib/Body Elements/Spherical Solid  GraphicAmbientColor=[0.15 0.15 0.15 1.0]  BasedOnType=Density  CenterOfMass=[0 0 0]  CenterOfMassUnits=m  GraphicDiffuseColor=[0.5 0.5 0.5]  Density=0.01  DensityUnits=kg/m^3  DoExposeReferenceFrame=on  GraphicEmissiveColor=[0.0 0.0 0.0 1.0]  ExportEntireGeometry=on  SerializedExposedGeometries=<ExposedGeometries><ExposedGeometry><RawGeometryId>entire</RawGeometryId><ExposedGeometryId>G</ExposedGeometryId></ExposedGeometry></ExposedGeometries>  SerializedFrames=<Frames/>  MarkerShape=Sphere  MarkerSize=10  GraphicType=FromGeometry  InertiaType=CalculateFromGeometry  Mass=1  MassUnits=kg  MomentsOfInertia=[1 1 1]  MomentsOfInertiaUnits=kg*m^2  GraphicOpacity=0  ProductsOfInertia=[0 0 0]  ProductsOfInertiaUnits=kg*m^2  GraphicShininess=75  GraphicSpecularColor=[0.5 0.5 0.5 1.0]  SphereRadius=0.1  SphereRadiusUnits=m  GraphicVisPropType=SimpleVisualProperties
  Transform Sensor : sm_lib/Frames and Transforms/Transform Sensor  MeasurementFrame=World  SenseAngle=off  SenseAxis=off  SenseAngle1=off  SenseAngle2=off  SenseAngle3=off  SenseQ=off  SenseR=off  SenseOmegaX=off  SenseOmegaY=off  SenseOmegaZ=off  SenseOmega1=off  SenseOmega2=off  SenseOmega3=off  SenseQDot=off  SenseRDot=off  SenseAlphaX=off  SenseAlphaY=off  SenseAlphaZ=off  SenseAlpha1=off  SenseAlpha2=off  SenseAlpha3=off  SenseQDDot=off  SenseRDDot=off  SenseX=off  SenseY=off  SenseZ=off  SenseRad=off  SenseAzim=off  SenseDist=on  SenseInc=off  SenseXDot=off  SenseYDot=off  SenseZDot=off  SenseRadDot=off  SenseAzimDot=off  SenseDistDot=off  SenseIncDot=off  SenseXDDot=off  SenseYDDot=off  SenseZDDot=off  SenseRadDDot=off  SenseAzimDDot=off  SenseDistDDot=off  SenseIncDDot=off
  Reference Frame : PMIOPort  Side=Left
  Brick Geometry : PMIOPort  Port=2  Side=Right
  Brick Centre : PMIOPort  Port=3  Side=Right
  Corner Geometries : PMIOPort  Port=4  Side=Right
  Cube Distance : PMIOPort  Port=5  Side=Left
  connections:
  Bushing Joint/RConn1 -- Transform Sensor/RConn1 -- Brick Solid/RConn1
  Reference Frame/RConn1 -- Block Placement/LConn1
  Block Placement/RConn1 -- Block Rotation/LConn1
  Block Rotation/RConn1 -- Transform Sensor/LConn1 -- Bushing Joint/LConn1
  Brick Solid/LConn1 -- Anti-Rotation/LConn1
  Rigid Transform1/LConn1 -- Rigid Transform2/LConn1 -- Rigid Transform4/LConn1 -- Rigid Transform5/LConn1 -- Rigid Transform6/LConn1 -- Rigid Transform7/LConn1 -- Rigid Transform3/LConn1 -- Brick Centre/RConn1 -- Anti-Rotation/RConn1 -- Rigid Transform/LConn1
  Brick Solid/LConn2 -- Brick Geometry/RConn1
  Spherical Solid4/LConn1 -- Simscape Bus/LConn5
  Rigid Transform6/RConn1 -- Spherical Solid6/RConn1
  Spherical Solid6/LConn1 -- Simscape Bus/LConn7
  Spherical Solid2/LConn1 -- Simscape Bus/LConn3
  Spherical Solid1/LConn1 -- Simscape Bus/LConn2
  Spherical Solid/LConn1 -- Simscape Bus/LConn1
  Spherical Solid3/LConn1 -- Simscape Bus/LConn4
  Rigid Transform5/RConn1 -- Spherical Solid5/RConn1
  Rigid Transform/RConn1 -- Spherical Solid/RConn1
  Rigid Transform1/RConn1 -- Spherical Solid1/RConn1
  Rigid Transform4/RConn1 -- Spherical Solid4/RConn1
  Spherical Solid7/LConn1 -- Simscape Bus/LConn8
  Spherical Solid5/LConn1 -- Simscape Bus/LConn6
  Rigid Transform7/RConn1 -- Spherical Solid7/RConn1
  Rigid Transform2/RConn1 -- Spherical Solid2/RConn1
  Corner Geometries/RConn1 -- Simscape Bus/RConn1
  Rigid Transform3/RConn1 -- Spherical Solid3/RConn1
  Cube Distance/RConn1 -- Transform Sensor/RConn2

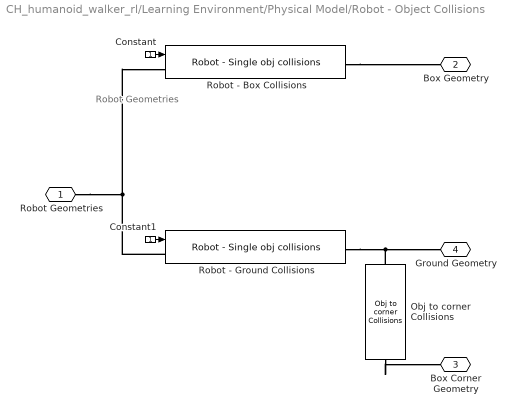
== system CH_humanoid_walker_rl/Learning Environment/Physical Model/Robot - Object Collisions ==
  note: Robot Geometries
  Constant : Constant
  Constant1 : Constant
  Obj to corner Collisions : CH_Library/Obj to corner Collisions  MatStatFric=0.05  MatDynFric=0.05  CritVel=1e-6  MatStiff=1e6  MatDamp=1e3  TransitionRegion=1e-4
  Robot - Box Collisions : CH_Library/Robot - Single obj collisions  SystemSampleTime=-1  VariantActivationTime=update diagram  Latency=0  AutoFrameSizeCalculation=off
  Robot - Ground Collisions : CH_Library/Robot - Single obj collisions  SystemSampleTime=-1  VariantActivationTime=update diagram  Latency=0  AutoFrameSizeCalculation=off
  Robot Geometries : PMIOPort  Side=Left
  Box Geometry : PMIOPort  Port=2  Side=Right
  Box Corner Geometry : PMIOPort  Port=3  Side=Right
  Ground Geometry : PMIOPort  Port=4  Side=Right
  wires:
  Constant/1 -> Robot - Box Collisions/1
  Constant1/1 -> Robot - Ground Collisions/1
  connections:
  Robot Geometries/RConn1 -- Robot - Box Collisions/LConn1 -- Robot - Ground Collisions/LConn1
  Robot - Box Collisions/RConn1 -- Box Geometry/RConn1
  Robot - Ground Collisions/RConn1 -- Ground Geometry/RConn1 -- Obj to corner Collisions/RConn1
  Obj to corner Collisions/LConn1 -- Box Corner Geometry/RConn1
